simulink model "AtuadorNaoLinear"  (R2024a)
settings: Solver=FixedStepAuto  StartTime=0.0  StopTime=tf  FixedStep=step_modelo  RelTol=1e-3
undefined symbols (not defined in the file or in its folder): Fn, rb, step_modelo
libraries: simulink x1
settings Model: PacingRate=1000  Creator=rodri  LastModifiedBy=rodri
settings DataIOCC: SaveOutput=off  SaveTime=off
settings RTWCC: GPUComputeCapability=3.5

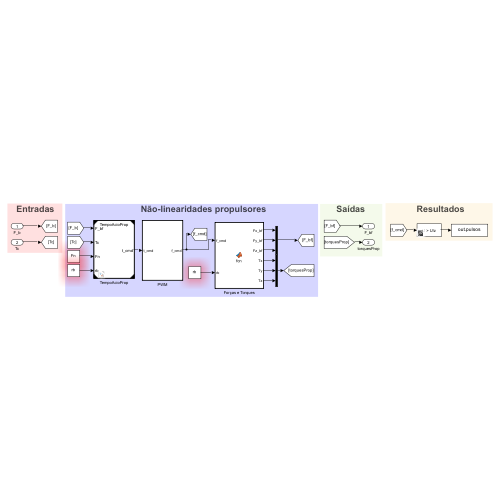
[thumbnail: Simulink's stored preview of the top-level diagram]
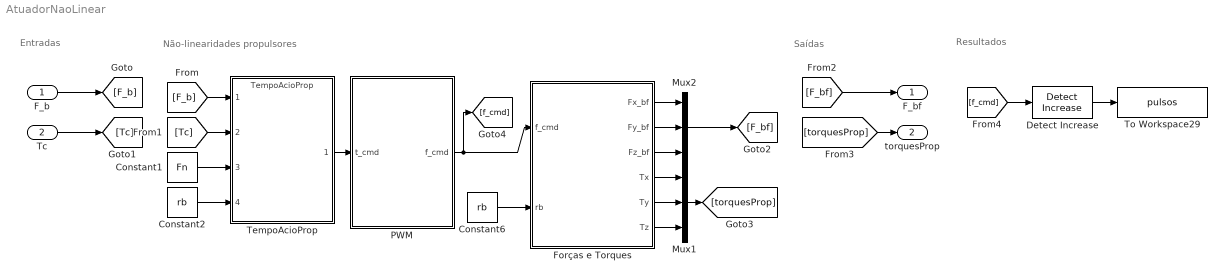
== system AtuadorNaoLinear ==
  note: Não-linearidades propulsores
  note: Saídas
  note: Entradas
  note: Resultados
  F_b : Inport
  Tc : Inport  Port=2
  Constant1 : Constant  Value=Fn  SampleTime=-1
  Constant2 : Constant  Value=rb  SampleTime=-1
  Constant6 : Constant  Value=rb  SampleTime=-1
  Detect Increase : simulink/Logic and Bit Operations/Detect Increase  vinit=0.0  OutDataTypeStr=uint8
  Forças e Torques : MATLAB Function  TreatAsAtomicUnit=on
  Mux1 : Mux  Inputs=3
  Mux2 : Mux  Inputs=3
  PWM : Subsystem  TreatAsAtomicUnit=on
  TempoAcioProp : ModelReference  ModelNameDialog=TempoAcioProp.slx  ModelReferenceVersion=3.1
  To Workspace29 : ToWorkspace  VariableName=pulsos  SampleTime=-1
      settings: Save2DSignal=2-D array (concatenate along first dimension)
  F_bf : Outport  OutDataTypeStr=double  PortDimensions=3
  torquesProp : Outport  Port=2  OutDataTypeStr=double  PortDimensions=3
  wires:
  Forças e Torques/4(Tx) -> Mux1/1
  Forças e Torques/1(Fx_bf) -> Mux2/1
  Constant2/1 -> TempoAcioProp/4
  Constant1/1 -> TempoAcioProp/3
  Forças e Torques/5(Ty) -> Mux1/2
  Constant6/1 -> Forças e Torques/2(rb)
  Forças e Torques/3(Fz_bf) -> Mux2/3
  Forças e Torques/6(Tz) -> Mux1/3
  Forças e Torques/2(Fy_bf) -> Mux2/2
  TempoAcioProp/1 -> PWM/1(t_cmd)
  F_b/1 -> [F_b]
  Tc/1 -> [Tc]
  [F_b] -> TempoAcioProp/1
  [Tc] -> TempoAcioProp/2
  Mux2/1 -> [F_bf]
  Mux1/1 -> [torquesProp]
  [F_bf] -> F_bf/1
  [torquesProp] -> torquesProp/1
  PWM/1(f_cmd) -> Forças e Torques/1(f_cmd), [f_cmd]
  [f_cmd] -> Detect Increase/1
  Detect Increase/1 -> To Workspace29/1

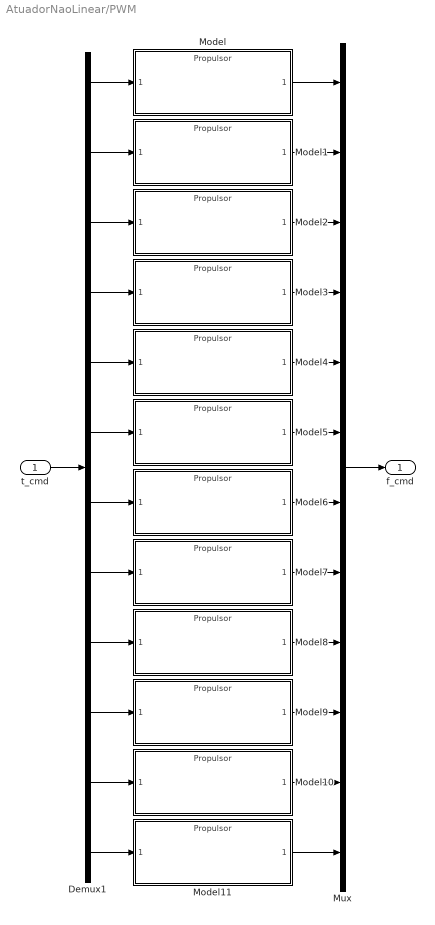
== system AtuadorNaoLinear/PWM ==
  t_cmd : Inport  SampleTime=step_modelo
  Demux1 : Demux  Outputs=12
  Model{,1..11} (12 alike) : ModelReference  ModelNameDialog=Propulsor.slx  ModelReferenceVersion=2.18
  Mux : Mux  Inputs=12
  f_cmd : Outport
  wires:
  Model4/1 -> Mux/5
  Model7/1 -> Mux/8
  Demux1/8 -> Model7/1
  Demux1/7 -> Model6/1
  Model11/1 -> Mux/12
  Model1/1 -> Mux/2
  Demux1/10 -> Model9/1
  Demux1/9 -> Model8/1
  Demux1/4 -> Model3/1
  Model2/1 -> Mux/3
  Demux1/5 -> Model4/1
  Mux/1 -> f_cmd/1
  t_cmd/1 -> Demux1/1
  Demux1/3 -> Model2/1
  Model5/1 -> Mux/6
  Demux1/6 -> Model5/1
  Demux1/2 -> Model1/1
  Model3/1 -> Mux/4
  Demux1/12 -> Model11/1
  Demux1/11 -> Model10/1
  Model8/1 -> Mux/9
  Model6/1 -> Mux/7
  Model10/1 -> Mux/11
  Model9/1 -> Mux/10
  Demux1/1 -> Model/1
  Model/1 -> Mux/1

== matlab function AtuadorNaoLinear/Forças e Torques ==
  data: f_cmd input; Fx_bf output; Fy_bf output; Fz_bf output; Tx output; Ty output; Tz output; rb input
function [Fx_bf,Fy_bf,Fz_bf,Tx,Ty,Tz] = fcn(f_cmd,rb)

f1 = f_cmd(1);
f2 = f_cmd(2);
f3 = f_cmd(3);
f4 = f_cmd(4);
f5 = f_cmd(5);
f6 = f_cmd(6);
f7 = f_cmd(7);
f8 = f_cmd(8);
f9 = f_cmd(9);
f10 = f_cmd(10);
f11 = f_cmd(11);
f12 = f_cmd(12);

Fx_bf = f1+f2-f7-f8;
Fy_bf = -f3-f4+f9+f10;
Fz_bf = -f5-f6+f11+f12;
Tx = f5*rb-f6*rb-f11*rb+f12*rb;
Ty = -f1*rb+f2*rb+f7*rb-f8*rb;
Tz = -f3*rb+f4*rb+f9*rb-f10*rb;


% A = [Fn Fn 0 0 0 0 -Fn -Fn 0 0 0 0
%     0 0 -Fn -Fn 0 0 0 0 Fn Fn 0 0
%     0 0 0 0 -Fn -Fn 0 0 0 0 Fn Fn
%     0 0 0 0 Tn -Tn 0 0 0 0 -Tn Tn
%     -Tn Tn 0 0 0 0 Tn -Tn 0 0 0 0
%     0 0 -Tn Tn 0 0 0 0 Tn -Tn 0 0];
